simulink model "CircuitoPi"  (R2015a)
settings: Solver=ode45  StartTime=0.0  StopTime=10/60  RelTol=1e-3
libraries: powerlib x16, powerlib_meascontrol x5
settings Model: Creator=note  LastModifiedBy=felip

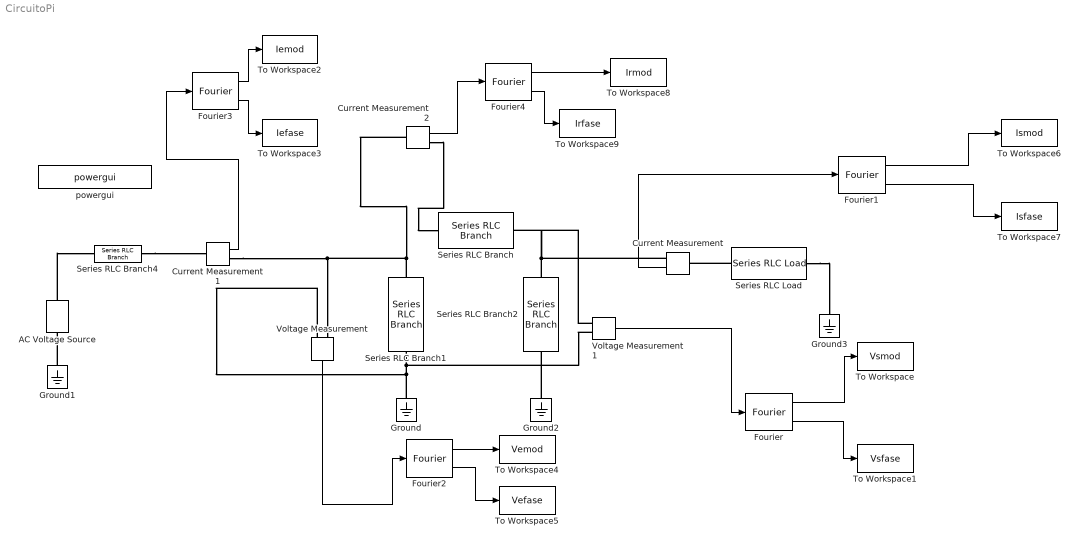
== system CircuitoPi ==
  AC Voltage Source : powerlib/Electrical Sources/AC Voltage Source  Amplitude=187794.2136  Phase=0  Frequency=60  SampleTime=0  Measurements=None
  Current Measurement : powerlib/Measurements/Current Measurement  PhasorSimulation=off  OutputType=Complex  PSBequivalent=0
  Current Measurement1 : powerlib/Measurements/Current Measurement  PhasorSimulation=off  OutputType=Complex  PSBequivalent=0
  Current Measurement2 : powerlib/Measurements/Current Measurement  PhasorSimulation=off  OutputType=Complex  PSBequivalent=0
  Fourier{,1..4} (5 alike) : powerlib_meascontrol/Measurements/Fourier  Freq=60  n=1  InInit=[0, 0]  Ts=0
  Ground{,1..3} (4 alike) : powerlib/Elements/Ground  LConnTagsString=a
  Series RLC Branch : powerlib/Elements/Series RLC Branch  LConnTagsString=__new0  RConnTagsString=__new0  BranchType=RL  Resistance=5  Inductance=129.45e-3  SetiL0=off  InitialCurrent=0  Capacitance=0  Setx0=off  InitialVoltage=0  Measurements=None
  Series RLC Branch1 : powerlib/Elements/Series RLC Branch  LConnTagsString=__new0  RConnTagsString=__new0  BranchType=C  Resistance=0  Inductance=0  SetiL0=off  InitialCurrent=0  Capacitance=(894.19/2)*10^(-9)  Setx0=off  InitialVoltage=0  Measurements=None
  Series RLC Branch2 : powerlib/Elements/Series RLC Branch  LConnTagsString=__new0  RConnTagsString=__new0  BranchType=C  Resistance=0  Inductance=0  SetiL0=off  InitialCurrent=0  Capacitance=(894.19/2)*10^(-9)  Setx0=off  InitialVoltage=0  Measurements=None
  Series RLC Branch4 : powerlib/Elements/Series RLC Branch  LConnTagsString=__new0  RConnTagsString=__new0  BranchType=R  Resistance=0.5  Inductance=1e-3  SetiL0=off  InitialCurrent=0  Capacitance=1e-6  Setx0=off  InitialVoltage=0  Measurements=None
  Series RLC Load : powerlib/Elements/Series RLC Load  LConnTagsString=a  RConnTagsString=__new0  NominalVoltage=230*10^3/sqrt(3)  NominalFrequency=60  ActivePower=0.8*140*10^6  InductivePower=0  CapacitivePower=0  Setx0=off  InitialVoltage=0  SetiL0=off  InitialCurrent=0  Measurements=None
  To Workspace : ToWorkspace  VariableName=Vsmod  SampleTime=-1
  To Workspace1 : ToWorkspace  VariableName=Vsfase  SampleTime=-1
  To Workspace2 : ToWorkspace  VariableName=Iemod  SampleTime=-1
  To Workspace3 : ToWorkspace  VariableName=Iefase  SampleTime=-1
  To Workspace4 : ToWorkspace  VariableName=Vemod  SampleTime=-1
  To Workspace5 : ToWorkspace  VariableName=Vefase  SampleTime=-1
  To Workspace6 : ToWorkspace  VariableName=Ismod  SampleTime=-1
  To Workspace7 : ToWorkspace  VariableName=Isfase  SampleTime=-1
  To Workspace8 : ToWorkspace  VariableName=Irmod  SampleTime=-1
  To Workspace9 : ToWorkspace  VariableName=Irfase  SampleTime=-1
  Voltage Measurement : powerlib/Measurements/Voltage Measurement  PhasorSimulation=off  OutputType=Complex  PSBequivalent=0
  Voltage Measurement1 : powerlib/Measurements/Voltage Measurement  PhasorSimulation=off  OutputType=Complex  PSBequivalent=0
  powergui : powerlib/powergui  SimulationMode=Discrete  SolverType=Tustin  SampleTime=50e-6  frequency=60  SPID=off  DisableSnubberDevices=off  DisableRonSwitches=off  DisableVfSwitches=off  SwTol=0  DisplayEquations=off  Interpol=off  methode=off  Ts=0  FunctionMessages=off  echomessages=off  HookPort=off  EnableUseOfTLC=off  x0status=steady  frequencyindice=60  Pbase=100e6  ErrMax=1e-4  Iterations=50  UnitsV=kV  UnitsW=MW  buscounter=0  RestoreLinks=warning  ResistiveCurrentMeasurement=off  Frange=[0:2:500]  Ylog=off  Xlog=on  ShowGrid=off  save=off  variable=ZData  structure=0  ZoomFFT=on  StartTime=0.0  cycles=1  DisplayStyle=1  fundamental=60  FreqAxis=off  MaxFrequency=1000  frequencyindicesteady=1  RmsSteady=2  display=off
  wires:
  Voltage Measurement1/1 -> Fourier/1
  Fourier/1 -> To Workspace/1
  Fourier/2 -> To Workspace1/1
  Current Measurement/1 -> Fourier1/1
  Voltage Measurement/1 -> Fourier2/1
  Current Measurement1/1 -> Fourier3/1
  Fourier3/1 -> To Workspace2/1
  Fourier3/2 -> To Workspace3/1
  Fourier2/1 -> To Workspace4/1
  Fourier2/2 -> To Workspace5/1
  Fourier1/1 -> To Workspace6/1
  Fourier1/2 -> To Workspace7/1
  Current Measurement2/1 -> Fourier4/1
  Fourier4/1 -> To Workspace8/1
  Fourier4/2 -> To Workspace9/1
  connections:
  Series RLC Branch1/RConn1 -- Current Measurement1/RConn1 -- Voltage Measurement/LConn1 -- Current Measurement2/LConn1
  Series RLC Branch2/RConn1 -- Voltage Measurement1/LConn1 -- Series RLC Branch/RConn1 -- Current Measurement/RConn1
  Ground/LConn1 -- Voltage Measurement1/LConn2 -- Series RLC Branch1/LConn1 -- Voltage Measurement/LConn2
  Ground1/LConn1 -- AC Voltage Source/LConn1
  Series RLC Load/RConn1 -- Ground3/LConn1
  Series RLC Load/LConn1 -- Current Measurement/LConn1
  Ground2/LConn1 -- Series RLC Branch2/LConn1
  AC Voltage Source/RConn1 -- Series RLC Branch4/LConn1
  Series RLC Branch4/RConn1 -- Current Measurement1/LConn1
  Current Measurement2/RConn1 -- Series RLC Branch/LConn1
